simulink model "task3_lab12"  (R2021a)
settings: Solver=VariableStepAuto  StartTime=0.0  StopTime=10.0  RelTol=1e-3
settings Model: Creator=reemb  LastModifiedBy=reemb

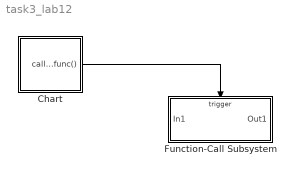
== system task3_lab12 ==
  Chart : Stateflow chart  TreatAsAtomicUnit=on
  Function-Call Subsystem : Subsystem  TreatAsAtomicUnit=on
  wires:
  Chart/1(call_my_func()) -> Function-Call Subsystem/Trigger

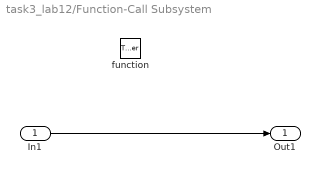
== system task3_lab12/Function-Call Subsystem ==
  In1 : Inport
  function : TriggerPort  TriggerType=function-call  VariantControl=(inherit)
  Out1 : Outport
  wires:
  In1/1 -> Out1/1

== stateflow chart task3_lab12/Chart ==
  state A
    entry: call_my_func()
  state B
  A -> B : after(1, sec)
  (default) -> A
  B -> A : after(1, sec)
  events: call_my_func output FUNCTION_CALL_EVENT
